simulink model "Communication_Testing"  (R2024a)
settings: Solver=FixedStepAuto  StartTime=0.0  StopTime=100  RelTol=1e-3  EnableMultiTasking=on
undefined symbols (not defined in the file or in its folder): CAN, FD
libraries: stmutilitieslib x29, simulink x25, stm32blockslib x11, canfdmsglib x7, stm32h7xxblockslib x3, dspstat3 x3, slpidlib x2
(part 2 of 2)

== system Communication_Testing/If Action Subsystem7 ==
  In1 : Inport
  Action Port : ActionPort  ActionPortLabel=case [ 235 ]:
  Out1 : Outport
  wires:
  In1/1 -> Out1/1

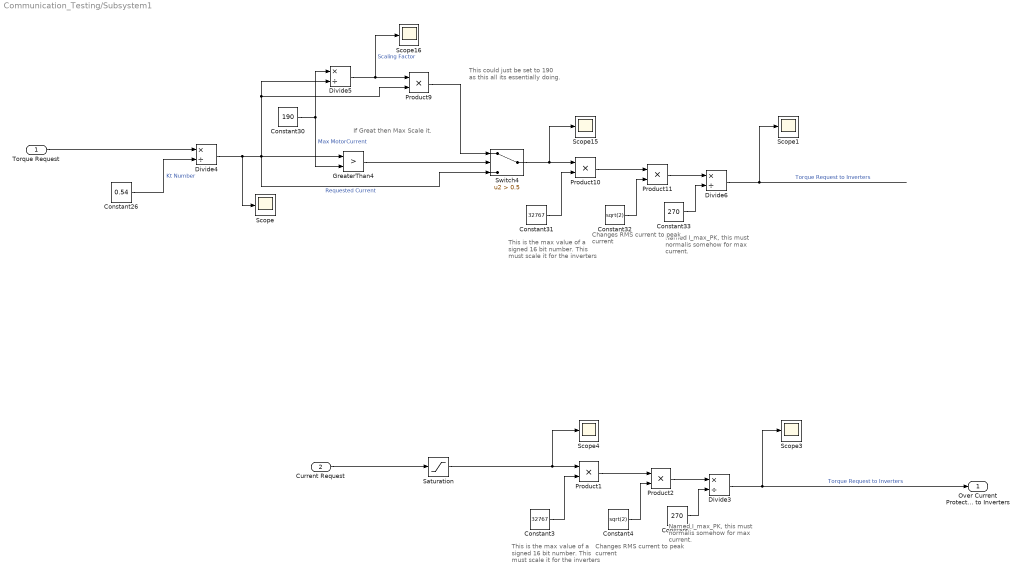
== system Communication_Testing/Subsystem1 ==
  note: This could just be set to 190 as this all its essentially doing.
  note: Named I_max_PK, this must normalis somehow for max current.
  note: Changes RMS current to peak current
  note: This is the max value of a signed 16 bit number. This must scale it for the inverters
  note: If Great then Max Scale it.
  note: Changes RMS current to peak current
  note: This is the max value of a signed 16 bit number. This must scale it for the inverters
  note: Named I_max_PK, this must normalis somehow for max current.
  Torque Request : Inport
  Current Request : Inport  Port=2
  Constant26 : Constant  Value=0.54
  Constant3 : Constant  Value=32767
  Constant30 : Constant  Value=190
  Constant31 : Constant  Value=32767
  Constant32 : Constant  Value=sqrt(2)
  Constant33 : Constant  Value=270
  Constant4 : Constant  Value=sqrt(2)
  Constant5 : Constant  Value=270
  Divide{3..6} (4 alike) : Product  Inputs=*/
  GreaterThan4 : RelationalOperator  Operator=>  OutDataTypeStr=boolean  RndMeth=Simplest  InputSameDT=off
  Product{1..2,9..11} (5 alike) : Product
  Saturation : Saturate  UpperLimit=190  LowerLimit=0
  Scope{,1,3..4,15..16} (6 alike) : Scope
  Switch4 : Switch  Criteria=u2 > Threshold  Threshold=0.5  SaturateOnIntegerOverflow=off  InputSameDT=off
  Over Current Protected Torque Request to Inverters : Outport
  wires:
  Constant31/1 -> Product10/2
  Product10/1 -> Product11/1
  Constant33/1 -> Divide6/2
  GreaterThan4/1 -> Switch4/2
  Divide5/1 -> Scope16/1, Product9/1  "Scaling Factor"
  Constant30/1 -> Divide5/1, GreaterThan4/2  "Max MotorCurrent"
  Product9/1 -> Switch4/1
  Divide4/1 -> Scope/1, Product9/2, Divide5/2, Switch4/3, GreaterThan4/1  "Requested Current"
  Constant26/1 -> Divide4/2  "Kt Number"
  Switch4/1 -> Product10/1, Scope15/1
  Constant32/1 -> Product11/2
  Product11/1 -> Divide6/1
  Torque Request/1 -> Divide4/1
  Divide6/1 -> Scope1/1  "Torque Request to Inverters"
  Product1/1 -> Product2/1
  Saturation/1 -> Product1/1, Scope4/1
  Divide3/1 -> Over Current Protected Torque Request to Inverters/1, Scope3/1  "Torque Request to Inverters"
  Constant4/1 -> Product2/2
  Constant5/1 -> Divide3/2
  Constant3/1 -> Product1/2
  Product2/1 -> Divide3/1
  Current Request/1 -> Saturation/1

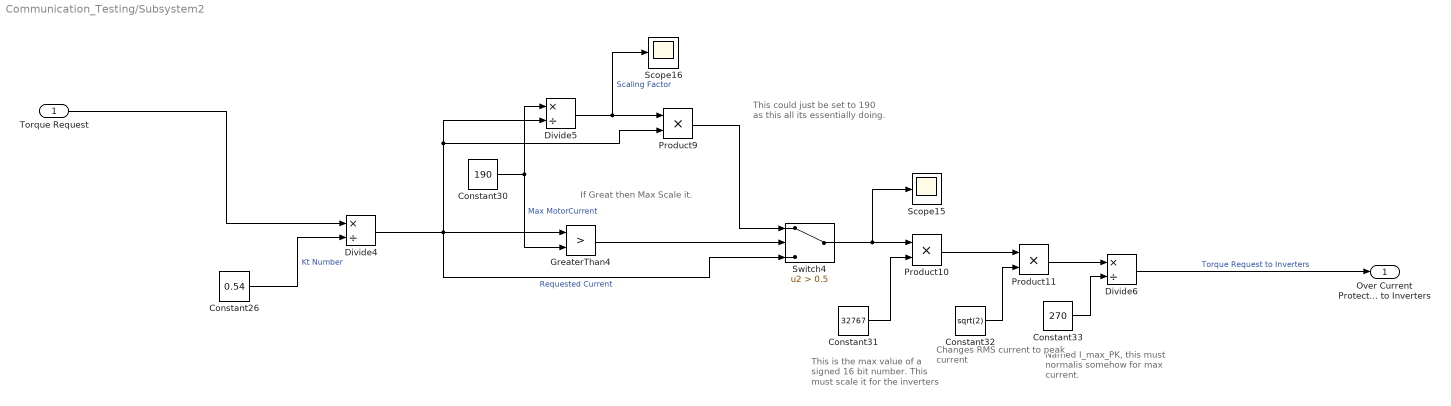
== system Communication_Testing/Subsystem2 ==
  note: This could just be set to 190 as this all its essentially doing.
  note: Named I_max_PK, this must normalis somehow for max current.
  note: Changes RMS current to peak current
  note: This is the max value of a signed 16 bit number. This must scale it for the inverters
  note: If Great then Max Scale it.
  Torque Request : Inport
  Constant26 : Constant  Value=0.54
  Constant30 : Constant  Value=190
  Constant31 : Constant  Value=32767
  Constant32 : Constant  Value=sqrt(2)
  Constant33 : Constant  Value=270
  Divide4 : Product  Inputs=*/
  Divide5 : Product  Inputs=*/
  Divide6 : Product  Inputs=*/
  GreaterThan4 : RelationalOperator  Operator=>  OutDataTypeStr=boolean  RndMeth=Simplest  InputSameDT=off
  Product10 : Product
  Product11 : Product
  Product9 : Product
  Scope15 : Scope
  Scope16 : Scope
  Switch4 : Switch  Criteria=u2 > Threshold  Threshold=0.5  SaturateOnIntegerOverflow=off  InputSameDT=off
  Over Current Protected Torque Request to Inverters : Outport
  wires:
  Constant31/1 -> Product10/2
  Product10/1 -> Product11/1
  Constant33/1 -> Divide6/2
  GreaterThan4/1 -> Switch4/2
  Divide5/1 -> Scope16/1, Product9/1  "Scaling Factor"
  Constant30/1 -> Divide5/1, GreaterThan4/2  "Max MotorCurrent"
  Product9/1 -> Switch4/1
  Divide4/1 -> Product9/2, Divide5/2, Switch4/3, GreaterThan4/1  "Requested Current"
  Constant26/1 -> Divide4/2  "Kt Number"
  Switch4/1 -> Product10/1, Scope15/1
  Constant32/1 -> Product11/2
  Product11/1 -> Divide6/1
  Torque Request/1 -> Divide4/1
  Divide6/1 -> Over Current Protected Torque Request to Inverters/1  "Torque Request to Inverters"

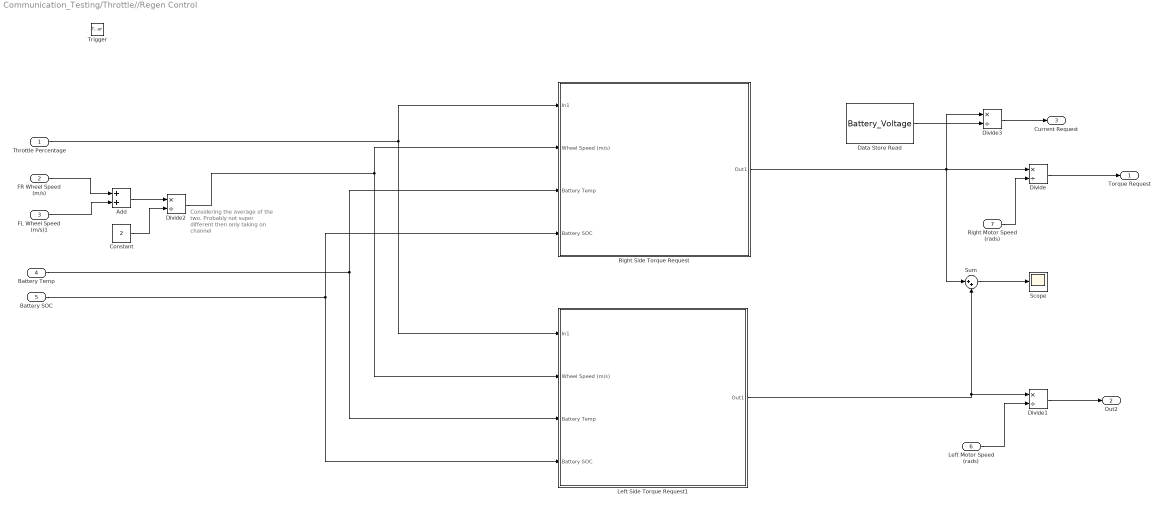
== system Communication_Testing/Throttle//Regen Control ==
  note: Considering the average of the two. Probably not super different then only taking on channel
  Throttle Percentage : Inport
  FR Wheel Speed (m/s) : Inport  Port=2
  FL Wheel Speed (m/s)1 : Inport  Port=3
  Battery Temp : Inport  Port=4
  Battery SOC : Inport  Port=5
  Left Motor Speed (rads) : Inport  Port=6
  Right Motor Speed (rads) : Inport  Port=7
  Trigger : TriggerPort  TriggerType=function-call  VariantControl=(inherit)
  Add : Sum
  Constant : Constant  Value=2
  Data Store Read : DataStoreRead  DataStoreName=Battery_Voltage  IndexOptions=Index vector (dialog)  Indices=1  OutputSizes=1
  Divide{,1..3} (4 alike) : Product  Inputs=*/
  Left Side Torque Request1 : Subsystem
  Right Side Torque Request : Subsystem
  Scope : Scope
  Sum : Sum  Inputs=|++
  Torque Request : Outport
  Out2 : Outport  Port=2
  Current Request : Outport  Port=3
  wires:
  Right Side Torque Request/1(Out1) -> Divide3/1, Divide/1, Sum/1
  Divide/1 -> Torque Request/1
  Left Motor Speed (rads)/1 -> Divide1/2
  Sum/1 -> Scope/1
  Left Side Torque Request1/1(Out1) -> Divide1/1, Sum/2
  Divide1/1 -> Out2/1
  Throttle Percentage/1 -> Left Side Torque Request1/1(In1), Right Side Torque Request/1(In1)
  Right Motor Speed (rads)/1 -> Divide/2
  Divide2/1 -> Left Side Torque Request1/2(Wheel Speed (m/s)), Right Side Torque Request/2(Wheel Speed (m/s))
  Battery Temp/1 -> Right Side Torque Request/3(Battery Temp), Left Side Torque Request1/3(Battery Temp)
  Battery SOC/1 -> Right Side Torque Request/4(Battery SOC), Left Side Torque Request1/4(Battery SOC)
  FR Wheel Speed (m/s)/1 -> Add/1
  FL Wheel Speed (m/s)1/1 -> Add/2
  Add/1 -> Divide2/1
  Constant/1 -> Divide2/2
  Data Store Read/1 -> Divide3/2
  Divide3/1 -> Current Request/1

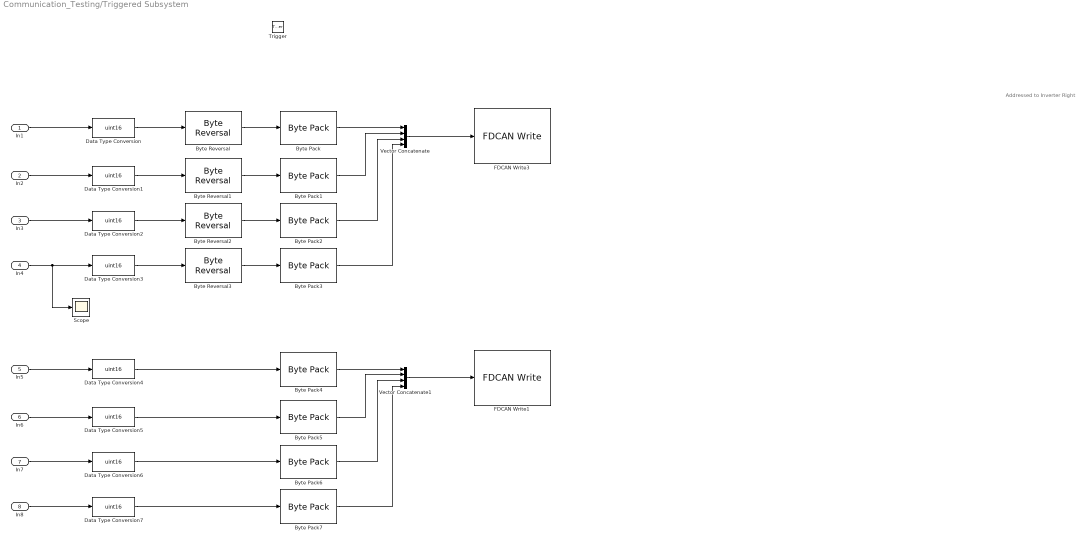
== system Communication_Testing/Triggered Subsystem ==
  note: Addressed to Inverter Right
  In1 : Inport
  In2 : Inport  Port=2
  In3 : Inport  Port=3
  In4 : Inport  Port=4
  In5 : Inport  Port=5
  In6 : Inport  Port=6
  In7 : Inport  Port=7
  In8 : Inport  Port=8
  Trigger : TriggerPort  TriggerType=function-call  VariantControl=(inherit)
  Byte Pack{,1..7} (8 alike) : stmutilitieslib/Byte Pack  datatypes={'uint16'}  byteAlign=1  blockPlatform=stm32f4discovery
  Byte Reversal{,1..3} (4 alike) : stmutilitieslib/Byte Reversal  numInp=1  blockPlatform=stm32f4discovery
  Data Type Conversion{,1..7} (8 alike) : DataTypeConversion  OutDataTypeStr=uint16  SaturateOnIntegerOverflow=off  RndMeth=Floor
  FDCAN Write1 : stm32blockslib/FDCAN Write  FDCANModule=FDCAN2  BlockMode=Transmit  OperationReadMode=Data  OperationWriteMode=Data  ReadSource=FIFO 0  BufferNumber=0  OutputTypeReadMode=Unpacked  DataFormatWriteMode=Raw data  CANFrameType=CAN  IdentifierTypeVia=Dialog  IdentifierType=Standard (11-bit identifier)  IdentifierVia=Dialog  Identifier=9  DataLengthVia=Dialog  DataLength=8  OutputIdType=off  IsBitRateSwitchingEnabled=off  TransmitRemoteFrame=off  OutputFrameType=off  OutputBRS=off  OutputRemoteFrame=off  OutputTxFifoLevel=off  OutputRxFifoLevel=off  OutputStatus=off  Timeout=1  SampleTime=-1
      settings: LibrarySourceBlock=stm32l5xxblockslib/FDCAN Write
  FDCAN Write3 : stm32blockslib/FDCAN Write  FDCANModule=FDCAN2  BlockMode=Transmit  OperationReadMode=Data  OperationWriteMode=Data  ReadSource=FIFO 0  BufferNumber=0  OutputTypeReadMode=Unpacked  DataFormatWriteMode=Raw data  CANFrameType=CAN  IdentifierTypeVia=Dialog  IdentifierType=Standard (11-bit identifier)  IdentifierVia=Dialog  Identifier=8  DataLengthVia=Dialog  DataLength=8  OutputIdType=off  IsBitRateSwitchingEnabled=off  TransmitRemoteFrame=off  OutputFrameType=off  OutputBRS=off  OutputRemoteFrame=off  OutputTxFifoLevel=off  OutputRxFifoLevel=off  OutputStatus=off  Timeout=1  SampleTime=-1
      settings: LibrarySourceBlock=stm32l5xxblockslib/FDCAN Write
  Scope : Scope
  Vector Concatenate : Concatenate  NumInputs=4
  Vector Concatenate1 : Concatenate  NumInputs=4
  wires:
  Byte Reversal/1 -> Byte Pack/1
  Byte Pack/1 -> Vector Concatenate/1
  Data Type Conversion/1 -> Byte Reversal/1
  In1/1 -> Data Type Conversion/1
  Byte Pack1/1 -> Vector Concatenate/2
  Byte Reversal1/1 -> Byte Pack1/1
  Data Type Conversion1/1 -> Byte Reversal1/1
  Byte Pack2/1 -> Vector Concatenate/3
  Byte Reversal2/1 -> Byte Pack2/1
  Data Type Conversion2/1 -> Byte Reversal2/1
  Byte Pack3/1 -> Vector Concatenate/4
  Byte Reversal3/1 -> Byte Pack3/1
  Data Type Conversion3/1 -> Byte Reversal3/1
  In2/1 -> Data Type Conversion1/1
  In3/1 -> Data Type Conversion2/1
  In4/1 -> Scope/1, Data Type Conversion3/1
  Vector Concatenate/1 -> FDCAN Write3/1
  Byte Pack6/1 -> Vector Concatenate1/3
  Data Type Conversion7/1 -> Byte Pack7/1
  Vector Concatenate1/1 -> FDCAN Write1/1
  Byte Pack5/1 -> Vector Concatenate1/2
  Byte Pack7/1 -> Vector Concatenate1/4
  Byte Pack4/1 -> Vector Concatenate1/1
  Data Type Conversion5/1 -> Byte Pack5/1
  Data Type Conversion6/1 -> Byte Pack6/1
  Data Type Conversion4/1 -> Byte Pack4/1
  In8/1 -> Data Type Conversion7/1
  In7/1 -> Data Type Conversion6/1
  In6/1 -> Data Type Conversion5/1
  In5/1 -> Data Type Conversion4/1

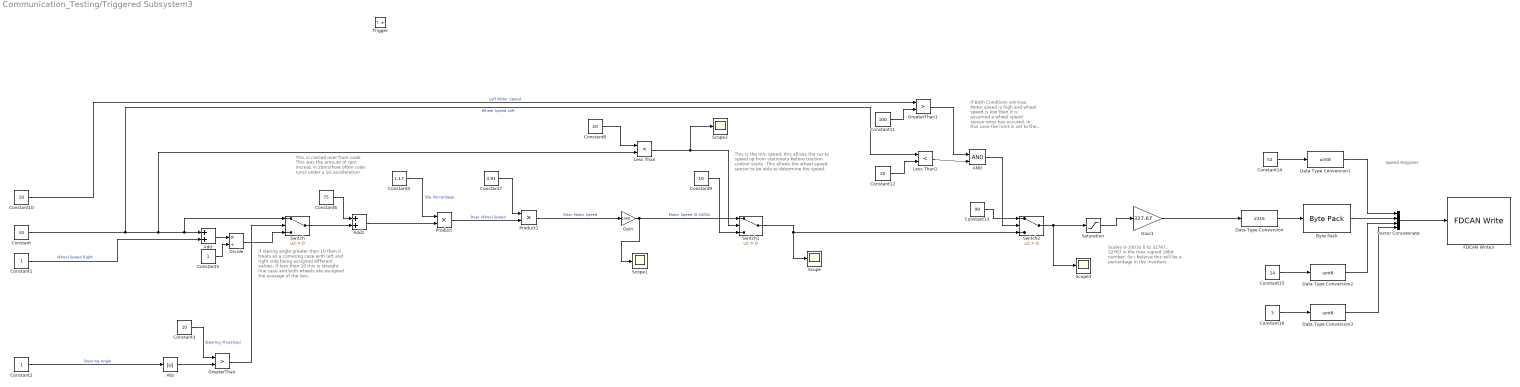
== system Communication_Testing/Triggered Subsystem3 ==
  note: This is the min speed, this allows the car to speed up from stationary before traction control starts, This allows the wheel speed sensor to be able to determine the speed.
  note: Scales 0-100 to 0 to 32767, 32767 is the max signed 16bit number, So i beleive this will be a percentage in the inverters
  note: If Both Conditons are true. Motor speed is high and wheel speed is low then it is assumed a wheel speed sensor error has occured. In this case the limit is set to the maximum.
  note: This is carried over from code. This was the amount of rpm increas in 20ms(how often code runs) under a 1G acceleration
  note: Speed Register
  note: if stering angle greater then 10 then it treats as a cornering case with left and right side being assigned different values. If less then 10 this is straight line case and both wheels are assigned the average of the two.
  Trigger : TriggerPort  TriggerType=function-call  VariantControl=(inherit)
  AND : Logic  IconShape=distinctive  AllPortsSameDT=off  OutDataTypeStr=boolean
  Abs : Abs  SaturateOnIntegerOverflow=off
  Add : Sum
  Add1 : Sum
  Byte Pack : stmutilitieslib/Byte Pack  datatypes={'int16'}  byteAlign=1  blockPlatform=stm32f4discovery
  Constant{,3,9..10} (4 alike) : Constant  Value=10
  Constant1 : Constant
  Constant11 : Constant  Value=100
  Constant12 : Constant  Value=20
  Constant13 : Constant  Value=99
  Constant14 : Constant  Value=52
  Constant15 : Constant  Value=14
  Constant16 : Constant  Value=3
  Constant2 : Constant
  Constant4 : Constant  Value=1.17
  Constant5 : Constant
  Constant6 : Constant  Value=75
  Constant7 : Constant  Value=3.91
  Constant8 : Constant  Value=20
  Data Type Conversion : DataTypeConversion  OutDataTypeStr=int16  SaturateOnIntegerOverflow=off  RndMeth=Floor
  Data Type Conversion1 : DataTypeConversion  OutDataTypeStr=uint8  SaturateOnIntegerOverflow=off  RndMeth=Floor
  Data Type Conversion2 : DataTypeConversion  OutDataTypeStr=uint8  SaturateOnIntegerOverflow=off  RndMeth=Floor
  Data Type Conversion3 : DataTypeConversion  OutDataTypeStr=uint8  SaturateOnIntegerOverflow=off  RndMeth=Floor
  Divide : Product  Inputs=*/
  FDCAN Write3 : stm32blockslib/FDCAN Write  FDCANModule=FDCAN2  BlockMode=Transmit  OperationReadMode=Data  OperationWriteMode=Data  ReadSource=FIFO 0  BufferNumber=0  OutputTypeReadMode=Unpacked  DataFormatWriteMode=Raw data  CANFrameType=CAN  IdentifierTypeVia=Dialog  IdentifierType=Standard (11-bit identifier)  IdentifierVia=Dialog  Identifier=210  DataLengthVia=Dialog  DataLength=5  OutputIdType=off  IsBitRateSwitchingEnabled=off  TransmitRemoteFrame=off  OutputFrameType=off  OutputBRS=off  OutputRemoteFrame=off  OutputTxFifoLevel=off  OutputRxFifoLevel=off  OutputStatus=off  Timeout=1  SampleTime=-1
      settings: LibrarySourceBlock=stm32l5xxblockslib/FDCAN Write
  Gain : Gain  Gain=1/60
  Gain1 : Gain  Gain=327.67
  GreaterThan : RelationalOperator  Operator=>  OutDataTypeStr=boolean  RndMeth=Simplest  InputSameDT=off
  GreaterThan1 : RelationalOperator  Operator=>  OutDataTypeStr=boolean  RndMeth=Simplest  InputSameDT=off
  Less Than : RelationalOperator  Operator=<  OutDataTypeStr=boolean  RndMeth=Simplest  InputSameDT=off
  Less Than1 : RelationalOperator  Operator=<  OutDataTypeStr=boolean  RndMeth=Simplest  InputSameDT=off
  Product : Product
  Product1 : Product
  Saturation : Saturate  UpperLimit=99  LowerLimit=0
  Scope{,1..3} (4 alike) : Scope
  Switch : Switch  Criteria=u2 > Threshold  SaturateOnIntegerOverflow=off  InputSameDT=off
  Switch1 : Switch  Criteria=u2 > Threshold  SaturateOnIntegerOverflow=off  InputSameDT=off
  Switch2 : Switch  Criteria=u2 > Threshold  SaturateOnIntegerOverflow=off  InputSameDT=off
  Vector Concatenate : Concatenate  NumInputs=4
  wires:
  Data Type Conversion/1 -> Byte Pack/1
  Switch2/1 -> Scope3/1, Saturation/1
  Less Than1/1 -> AND/2
  Gain1/1 -> Data Type Conversion/1
  Constant13/1 -> Switch2/1
  Data Type Conversion1/1 -> Vector Concatenate/1
  AND/1 -> Switch2/2
  Switch1/1 -> Switch2/3, Scope/1
  Data Type Conversion2/1 -> Vector Concatenate/3
  GreaterThan1/1 -> AND/1
  Constant8/1 -> Less Than/1
  Saturation/1 -> Gain1/1
  Constant11/1 -> GreaterThan1/2
  Less Than/1 -> Switch1/2, Scope2/1
  Gain/1 -> Switch1/1, Scope1/1  "Motor Speed (0-100%)"
  Constant16/1 -> Data Type Conversion3/1
  Product1/1 -> Gain/1  "Rear Motor Speed"
  Divide/1 -> Switch/3
  Constant15/1 -> Data Type Conversion2/1
  Add1/1 -> Product/2
  Constant9/1 -> Switch1/3
  Constant2/1 -> Abs/1  "Steering Angle"
  Constant10/1 -> GreaterThan1/1  "Left Motor Speed"
  Add/1 -> Divide/1
  Constant4/1 -> Product/1  "Slip Percentage"
  Product/1 -> Product1/2  "Rear Wheel Speed"
  Constant12/1 -> Less Than1/2
  Constant5/1 -> Divide/2
  Constant3/1 -> GreaterThan/1  "Steering Threshold"
  Byte Pack/1 -> Vector Concatenate/2
  Switch/1 -> Add1/2
  Constant7/1 -> Product1/1
  Constant1/1 -> Add/2  "Wheel Speed Right"
  GreaterThan/1 -> Switch/2
  Constant6/1 -> Add1/1
  Constant14/1 -> Data Type Conversion1/1
  Constant/1 -> Less Than1/1, Less Than/2, Switch/1, Add/1  "Wheel Speed Left"
  Abs/1 -> GreaterThan/2
  Data Type Conversion3/1 -> Vector Concatenate/4
  Vector Concatenate/1 -> FDCAN Write3/1

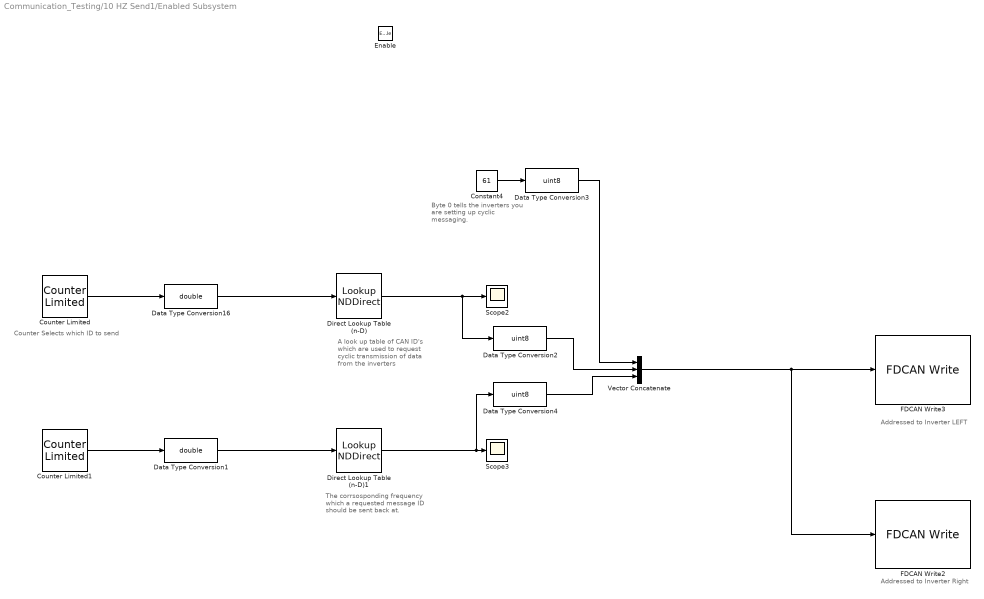
== system Communication_Testing/10 HZ Send1/Enabled Subsystem ==
  note: The corrsosponding frequency which a requested message ID should be sent back at.
  note: A look up table of CAN ID's which are used to request cyclic transmission of data from the inverters
  note: Byte 0 tells the inverters you are setting up cyclic messaging.
  note: Addressed to Inverter LEFT
  note: Counter Selects which ID to send
  note: Addressed to Inverter Right
  Enable : EnablePort
  Constant4 : Constant  Value=61
  Counter Limited : simulink/Sources/Counter Limited  uplimit=5  tsamp=-1
  Counter Limited1 : simulink/Sources/Counter Limited  uplimit=5  tsamp=-1
  Data Type Conversion1 : DataTypeConversion  OutDataTypeStr=double  SaturateOnIntegerOverflow=off  RndMeth=Floor
  Data Type Conversion16 : DataTypeConversion  OutDataTypeStr=double  SaturateOnIntegerOverflow=off  RndMeth=Floor
  Data Type Conversion2 : DataTypeConversion  OutDataTypeStr=uint8  SaturateOnIntegerOverflow=off  RndMeth=Floor
  Data Type Conversion3 : DataTypeConversion  OutDataTypeStr=uint8  SaturateOnIntegerOverflow=off  RndMeth=Floor
  Data Type Conversion4 : DataTypeConversion  OutDataTypeStr=uint8  SaturateOnIntegerOverflow=off  RndMeth=Floor
  Direct Lookup Table (n-D) : LookupNDDirect  NumberOfTableDimensions=1  Table=[235 74 168 73 95 138]
  Direct Lookup Table (n-D)1 : LookupNDDirect  NumberOfTableDimensions=1  Table=[235 74 168 73 95 138]
  FDCAN Write2 : stm32blockslib/FDCAN Write  FDCANModule=FDCAN2  BlockMode=Transmit  OperationReadMode=Data  OperationWriteMode=Data  ReadSource=FIFO 0  BufferNumber=0  OutputTypeReadMode=Unpacked  DataFormatWriteMode=Raw data  CANFrameType=CAN  IdentifierTypeVia=Dialog  IdentifierType=Standard (11-bit identifier)  IdentifierVia=Dialog  Identifier=529  DataLengthVia=Dialog  DataLength=3  OutputIdType=off  IsBitRateSwitchingEnabled=off  TransmitRemoteFrame=off  OutputFrameType=off  OutputBRS=off  OutputRemoteFrame=off  OutputTxFifoLevel=off  OutputRxFifoLevel=off  OutputStatus=off  Timeout=1  SampleTime=-1
      settings: LibrarySourceBlock=stm32l5xxblockslib/FDCAN Write
  FDCAN Write3 : stm32blockslib/FDCAN Write  FDCANModule=FDCAN2  BlockMode=Transmit  OperationReadMode=Data  OperationWriteMode=Data  ReadSource=FIFO 0  BufferNumber=0  OutputTypeReadMode=Unpacked  DataFormatWriteMode=Raw data  CANFrameType=CAN  IdentifierTypeVia=Dialog  IdentifierType=Standard (11-bit identifier)  IdentifierVia=Dialog  Identifier=528  DataLengthVia=Dialog  DataLength=3  OutputIdType=off  IsBitRateSwitchingEnabled=off  TransmitRemoteFrame=off  OutputFrameType=off  OutputBRS=off  OutputRemoteFrame=off  OutputTxFifoLevel=off  OutputRxFifoLevel=off  OutputStatus=off  Timeout=1  SampleTime=-1
      settings: LibrarySourceBlock=stm32l5xxblockslib/FDCAN Write
  Scope2 : Scope
  Scope3 : Scope
  Vector Concatenate : Concatenate  NumInputs=3
  wires:
  Direct Lookup Table (n-D)1/1 -> Data Type Conversion4/1, Scope3/1
  Data Type Conversion1/1 -> Direct Lookup Table (n-D)1/1
  Data Type Conversion16/1 -> Direct Lookup Table (n-D)/1
  Direct Lookup Table (n-D)/1 -> Data Type Conversion2/1, Scope2/1
  Counter Limited1/1 -> Data Type Conversion1/1
  Counter Limited/1 -> Data Type Conversion16/1
  Vector Concatenate/1 -> FDCAN Write2/1, FDCAN Write3/1
  Data Type Conversion3/1 -> Vector Concatenate/1
  Data Type Conversion4/1 -> Vector Concatenate/3
  Data Type Conversion2/1 -> Vector Concatenate/2
  Constant4/1 -> Data Type Conversion3/1

== system Communication_Testing/Function-Call Subsystem/If Action Subsystem1 ==
  In1 : Inport
  Action Port : ActionPort  ActionPortLabel=case [ 138 ]:
  Out1 : Outport
  wires:
  In1/1 -> Out1/1

== system Communication_Testing/Function-Call Subsystem/If Action Subsystem10 ==
  In1 : Inport
  Action Port : ActionPort  ActionPortLabel=case [ 168 ]:
  Out1 : Outport
  wires:
  In1/1 -> Out1/1

== system Communication_Testing/Function-Call Subsystem/If Action Subsystem11 ==
  In1 : Inport
  Action Port : ActionPort  ActionPortLabel=case [ 74 ]:
  Out1 : Outport
  wires:
  In1/1 -> Out1/1

== system Communication_Testing/Function-Call Subsystem/If Action Subsystem12 ==
  In1 : Inport
  Action Port : ActionPort  ActionPortLabel=case [ 235 ]:
  Out1 : Outport
  wires:
  In1/1 -> Out1/1

== system Communication_Testing/Function-Call Subsystem/If Action Subsystem2 ==
  In1 : Inport
  Action Port : ActionPort  ActionPortLabel=case [ 95 ]:
  Out1 : Outport
  wires:
  In1/1 -> Out1/1

== system Communication_Testing/Function-Call Subsystem/If Action Subsystem3 ==
  In1 : Inport
  Action Port : ActionPort  ActionPortLabel=case [ 73 ]:
  Out1 : Outport
  wires:
  In1/1 -> Out1/1

== system Communication_Testing/Function-Call Subsystem/If Action Subsystem4 ==
  In1 : Inport
  Action Port : ActionPort  ActionPortLabel=case [ 168 ]:
  Out1 : Outport
  wires:
  In1/1 -> Out1/1

== system Communication_Testing/Function-Call Subsystem/If Action Subsystem5 ==
  In1 : Inport
  Action Port : ActionPort  ActionPortLabel=case [ 74 ]:
  Out1 : Outport
  wires:
  In1/1 -> Out1/1

== system Communication_Testing/Function-Call Subsystem/If Action Subsystem6 ==
  In1 : Inport
  Action Port : ActionPort  ActionPortLabel=case [ 235 ]:
  Out1 : Outport
  wires:
  In1/1 -> Out1/1

== system Communication_Testing/Function-Call Subsystem/If Action Subsystem7 ==
  In1 : Inport
  Action Port : ActionPort  ActionPortLabel=case [ 138 ]:
  Out1 : Outport
  wires:
  In1/1 -> Out1/1

== system Communication_Testing/Function-Call Subsystem/If Action Subsystem8 ==
  In1 : Inport
  Action Port : ActionPort  ActionPortLabel=case [ 95 ]:
  Out1 : Outport
  wires:
  In1/1 -> Out1/1

== system Communication_Testing/Function-Call Subsystem/If Action Subsystem9 ==
  In1 : Inport
  Action Port : ActionPort  ActionPortLabel=case [ 73 ]:
  Out1 : Outport
  wires:
  In1/1 -> Out1/1

== system Communication_Testing/Function-Call Subsystem2/Subsystem ==
  Constant2 : Constant
  Out1 : Outport
  wires:
  Constant2/1 -> Out1/1

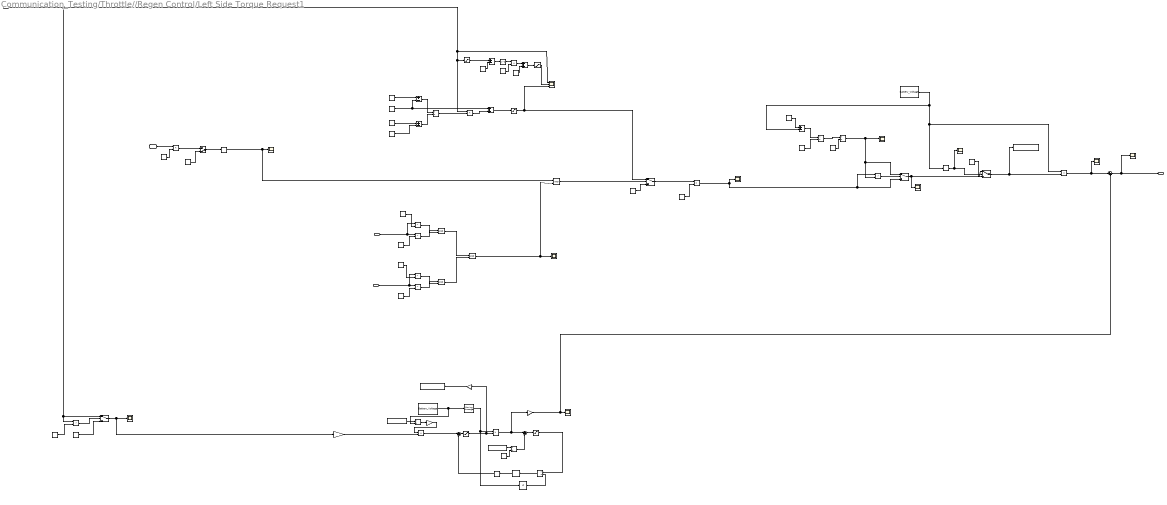
== system Communication_Testing/Throttle//Regen Control/Left Side Torque Request1 ==
  note: Divide by two as the global power is the power limit for the whole vehicle, then need the left and right side power limits
  note: Halveing as this is the permissable for left/right side inverter
  note: If Conditions are not fulfilled charge current is set to zero
  note: This function was made in Desmos. Adjusted to meet cross over and start of rise
  note: Throttle pedal to regen percentage request
  note: Power Limiting to maintatin Power Limit of Less then 80 Kw
  note: Inverting as this is a discharge current
  note: throttle output enabled when less then 20% actuation, this will be used for regen
  note: If Battery Voltage greater then 590 Charge Current is set to zero
  note: Throttle Mapping to Regen Percentage
  note: Limiting the input range
  note: Speed Threshold, Regen enabled above 5km/h
  note: Max Charge Current, Regen is scalled 0-100%. Current wants to be 0 -130 amps, therfore scale by 1.3. 600V*130amps = 70kw, Then divide by two for left and right motor Control
  note: Hysterisies Control
  note: Inverting as this is a discharge current
  note: Battery Checks
  note: This is the threshold for when drive torque is requested, Regen is requested for less then 20%, and throttle is applied for greater then 22%, This gives a 2% deadband
  note: If Requested Charge current is greater then permissable charge current then switch to permisable
  In1 : Inport
  Wheel Speed (m/s) : Inport  Port=2
  Battery Temp : Inport  Port=3
  Battery SOC : Inport  Port=4
  AND{,1..3} (4 alike) : Logic  IconShape=distinctive  AllPortsSameDT=off  OutDataTypeStr=boolean
  Add2 : Sum
  Add3 : Sum
  Compare To Constant : simulink/Logic and Bit Operations/Compare To Constant  relop=>  const=5  OutDataTypeStr=boolean
  Constant : Constant  Value=2
  Constant{7,10..11,21,28} (5 alike) : Constant  Value=0
  Constant12 : Constant  Value=6
  Constant15 : Constant  Value=0.01
  Constant16 : Constant  Value=50
  Constant17 : Constant  Value=10
  Constant18 : Constant  Value=90
  Constant19 : Constant  Value=5
  Constant2 : Constant  Value=3.6
  Constant20 : Constant  Value=580
  Constant26 : Constant  Value=2
  Constant27 : Constant  Value=22
  Constant3 : Constant  Value=20
  Constant4 : Constant  Value=10
  Constant5 : Constant  Value=100
  Constant6 : Constant  Value=20
  Constant9 : Constant  Value=0.25
  Data Store Read : DataStoreRead  DataStoreName=Battery_Voltage  IndexOptions=Index vector (dialog)  Indices=1  OutputSizes=1
  Data Store Read1 : DataStoreRead  DataStoreName=Battery_Voltage  IndexOptions=Index vector (dialog)  Indices=1  OutputSizes=1
  Data Store Read2 : DataStoreRead  DataStoreName=Global_Power_Limit  IndexOptions=Index vector (dialog)  Indices=1  OutputSizes=1
  Data Store Read3 : DataStoreRead  DataStoreName=Global_Power_Limit  IndexOptions=Index vector (dialog)  Indices=1  OutputSizes=1
  Data Store Write : DataStoreWrite  DataStoreName=Left_Sim_Regen_Current  IndexOptions=Index vector (dialog)  Indices=1  OutputSizes=1
  Data Store Write1 : DataStoreWrite  DataStoreName=Left_Sim_Discharge_Current  IndexOptions=Index vector (dialog)  Indices=1  OutputSizes=1
  Discrete PID Controller1 : slpidlib/PID Controller  Controller=PID  Form=Parallel  TimeDomain=Discrete-time  UseExternalTs=off  SampleTime=-1  IntegratorMethod=Forward Euler  FilterMethod=Forward Euler  ControllerParametersSource=internal  P=0.000544217300579932  I=0.544217300579932  UseKiTs=on  D=0  UseExternalDerivativeSource=off  N=100  UseFilter=on  TunerSelectOption=Transfer Function Based (PID Tuner App)  InitialConditionSource=internal  InitialConditionForIntegrator=10  InitialConditionForFilter=0  DifferentiatorICPrevScaledInput=0  ExternalReset=none  TrackingMode=off  Kt=1  LimitOutput=off  SatLimitsSource=internal  UpperSaturationLimit=inf  LowerSaturationLimit=-inf  LinearizeAsGain=off  AntiWindupMode=none  Kb=1  LimitIntegrator=off  UpperIntegratorSaturationLimit=inf  LowerIntegratorSaturationLimit=-inf  POutMin=[]  POutMax=[]  IOutMin=[]  IOutMax=[]  DOutMin=[]  DOutMax=[]  NOutMin=[]  NOutMax=[]  SumOutMin=[]  SumOutMax=[]  SaturationOutMin=[]  SaturationOutMax=[]  PParamMin=[]  PParamMax=[]  IParamMin=[]  IParamMax=[]  DParamMin=[]  DParamMax=[]  NParamMin=[]  NParamMax=[]  KbParamMin=[]  KbParamMax=[]  KtParamMin=[]  KtParamMax=[]  KbOutMin=[]  KbOutMax=[]  KtOutMin=[]  KtOutMax=[]  IntegratorOutMin=[]  IntegratorOutMax=[]  FilterOutMin=[]  FilterOutMax=[]  SumI1OutMin=[]  SumI1OutMax=[]  SumI2OutMin=[]  SumI2OutMax=[]  SumI3OutMin=[]  SumI3OutMax=[]  SumI4OutMin=[]  SumI4OutMax=[]  SumDOutMin=[]  SumDOutMax=[]  DifferentiatorOutMin=[]  DifferentiatorOutMax=[]  FilterDiffOutCoefMin=[]  FilterDiffOutCoefMax=[]  ReciprocalOutMin=[]  ReciprocalOutMax=[]  SumDenOutMin=[]  SumDenOutMax=[]  SumNumOutMin=[]  SumNumOutMax=[]  DivideOutMin=[]  DivideOutMax=[]  UdiffTsProdOutMin=[]  UdiffTsProdOutMax=[]  NTsProdOutMin=[]  NTsProdOutMax=[]  UintegralTsProdOutMin=[]  UintegralTsProdOutMax=[]  UngainTsProdOutMin=[]  UngainTsProdOutMax=[]  ClampingZeroOutDataTypeStr=Inherit: Inherit via back propagation  ClampingZeroOutMin=[]  ClampingZeroOutMax=[]  FilterDenConstantOutDataTypeStr=Inherit: Inherit via back propagation  FilterDenConstantOutMin=[]  FilterDenConstantOutMax=[]  PCopyOutDataTypeStr=Inherit: Inherit via back propagation  PCopyOutMin=[]  PCopyOutMax=[]  NCopyOutDataTypeStr=Inherit: Inherit via back propagation  NCopyOutMin=[]  NCopyOutMax=[]  IntegratorContinuousStateAttributes=''  IntegratorStateMustResolveToSignalObject=off  IntegratorRTWStateStorageClass=Auto  FilterContinuousStateAttributes=''  FilterStateMustResolveToSignalObject=off  FilterRTWStateStorageClass=Auto  ParallelPVariant=InternalParameters  IdealPVariant=Disabled  IVariant=InternalParameters  DVariant=InternalParameters  IntegratorVariant=Discrete  SatVariant=Disabled  AWVariant=Passthrough  PCopyVariant=Disabled  TRVariant=Disabled  FdbkBlocksVariant=Forward  IdealPFdbkVariant=Disabled  SatFdbkVariant=Disabled  DerivativeFilterVariant=ForwardEulerFilter  NVariant=InternalParameters  NCopyVariant=Disabled  FilterICVariant=InternalICsFilter  IntegratorICVariant=InternalICs  ExternalResetVariant=Disabled  TRSumVariant=Passthrough  SumFdbkVariant=Disabled  SumVariant=Sum_PID  TsampFilterVariant=InternalTs  TsampNgainVariant=Passthrough  TsampIntegralVariant=Disabled_SignalSpec  ExternalSaturationOutDataTypeStr=Inherit: Same as second input  DerivativeSourceVariant=ErrorSignal
      settings: LibrarySourceBlock=simulink/Discrete/Discrete PID Controller
  Divide{,1..5} (6 alike) : Product  Inputs=*/
  Gain : Gain  Gain=-1
  Gain1 : Gain  Gain=-1
  Gain2 : Gain  Gain=1/100
  Gain3 : Gain  Gain=1.1
  GreaterThan{,1..3} (4 alike) : RelationalOperator  Operator=>  OutDataTypeStr=boolean  RndMeth=Simplest  InputSameDT=off
  IC1 : InitialCondition  Value=600
  Less Than : RelationalOperator  Operator=<  OutDataTypeStr=boolean  RndMeth=Simplest  InputSameDT=off
  Less Than1 : RelationalOperator  Operator=<  OutDataTypeStr=boolean  RndMeth=Simplest  InputSameDT=off
  Manual Switch1 : ManualSwitch  CurrentSetting=0
  Memory1 : Memory  InitialCondition=14  InheritSampleTime=on
  Minus : Sum  Inputs=+-
  Moving Average : dspstat3/Moving Average  Method=Sliding window  ForgettingFactorPort=off  SpecifyWindowLength=on  WindowLength=10  OverlapLength=9  AllowArbitraryInputLength=off  ForgettingFactor=0.9  SimulateUsing=Interpreted execution
  Product{1..7} (7 alike) : Product
  Relay : Relay  OnSwitchValue=590  OffSwitchValue=585  OnOutputValue=0  OffOutputValue=1
  Saturation : Saturate  UpperLimit=100  LowerLimit=0
  Saturation1 : Saturate  UpperLimit=100  LowerLimit=0
  Saturation2 : Saturate  UpperLimit=20  LowerLimit=0
  Saturation3 : Saturate  UpperLimit=inf  LowerLimit=0
  Saturation5 : Saturate  UpperLimit=inf  LowerLimit=0
  Scale : Constant  Value=0.65
  Scope{,1,3,5,7..9,11,13..14} (10 alike) : Scope
  Scope2 : Scope  NumInputPorts=3
  Square : Math  Operator=square
  Subtract : Sum  Inputs=+-
  Subtract1 : Sum  Inputs=+-
  Subtract2 : Sum  Inputs=+-
  Sum : Sum  Inputs=|+-
  Sum1 : Sum  Inputs=|+-
  Sum3 : Sum  Inputs=|++
  Switch : Switch  Criteria=u2 > Threshold  SaturateOnIntegerOverflow=off  InputSameDT=off
  Switch1 : Switch  Criteria=u2 > Threshold  SaturateOnIntegerOverflow=off  InputSameDT=off
  Switch2 : Switch  Criteria=u2 > Threshold  Threshold=0.5  SaturateOnIntegerOverflow=off  InputSameDT=off
  Switch3 : Switch  Criteria=u2 > Threshold  SaturateOnIntegerOverflow=off  InputSameDT=off
  Out1 : Outport
  wires:
  Constant26/1 -> Divide4/2
  Product3/1 -> Add2/1
  Constant10/1 -> Add2/2
  Constant3/1 -> Subtract2/2
  AND/1 -> Switch/2
  Add3/1 -> Saturation/1  "Regen Request"
  GreaterThan2/1 -> Switch1/2
  Constant12/1 -> Manual Switch1/2
  GreaterThan1/1 -> AND2/1
  Constant21/1 -> Switch2/3
  In1/1 -> Switch3/1, GreaterThan3/1, Product2/1, Saturation2/1, Scope2/1  "Throttle Pedal"
  Constant11/1 -> Switch/3
  Switch3/1 -> Gain2/1, Scope14/1  "Throttle Percentage > 20"
  Product5/1 -> Sum1/1, Gain1/1  "Requested Discharge Power"
  Saturation/1 -> Switch/1, Scope2/3  "Linear Regen Map"
  Switch/1 -> Product4/1  "Requested Charge Current"
  Saturation1/1 -> Scope2/2  "Exponential Throttle Map"
  Gain1/1 -> Sum3/2, Scope5/1
  Constant27/1 -> GreaterThan3/2
  Constant20/1 -> Minus/1  "Max Battery Voltage using Regen"
  Constant5/1 -> Subtract/2, Add3/1  "Max Regen Percentage"
  Constant19/1 -> GreaterThan1/2  "Min Battery SOC"
  Subtract2/1 -> Square/1
  Product7/1 -> Scope13/1, Sum3/1  "Requested Charge Power"
  Subtract/1 -> Divide1/1
  Battery SOC/1 -> GreaterThan1/1, Less Than1/1  "Battery State of Charge"
  Moving Average/1 -> IC1/1, Product5/1
  Saturation3/1 -> Divide2/1  "Power Error"
  Manual Switch1/1 -> Compare To Constant/1
  Product1/1 -> Manual Switch1/1  "Speed (km/h)"
  Subtract1/1 -> Divide1/2
  Constant17/1 -> GreaterThan/2  "Min Battery Temp"
  Saturation5/1 -> Gain/1, Product5/2
  Divide3/1 -> Sum1/2
  Product6/1 -> Sum/1  "Current Request (0-75amps)"
  Constant28/1 -> Switch3/3
  Square/1 -> Product3/1
  Saturation2/1 -> Subtract2/1  "Exponential Throttle Map"
  Sum3/1 -> Out1/1, Scope11/1
  Constant16/1 -> Less Than/2  "Max Battery temp"
  GreaterThan3/1 -> Switch3/2
  Constant6/1 -> Subtract1/1  "Minimum Throttle Percentage"
  Constant9/1 -> Product3/2
  Add2/1 -> Saturation1/1
  Wheel Speed (m/s)/1 -> Product1/1  "Speed (m/s)"
  AND3/1 -> Scope3/1, AND/2  "Battery Logic"
  Divide/1 -> Divide4/1
  Compare To Constant/1 -> AND/1, Scope1/1
  Sum/1 -> Saturation5/1
  Constant18/1 -> Less Than1/2  "Max Battery SOC"
  Constant7/1 -> Subtract1/2  "Intial distance"
  AND2/1 -> AND3/2
  Memory1/1 -> Sum/2
  AND1/1 -> AND3/1
  Constant2/1 -> Product1/2
  Data Store Read1/1 -> Minus/2, Product7/1, Relay/1
  Constant4/1 -> Subtract/1  "Min Regen Percentage"
  Less Than1/1 -> AND2/2
  Minus/1 -> Divide/1  "Voltage Threshold to overcharge"
  GreaterThan/1 -> AND1/1
  Scale/1 -> Product4/2
  Sum1/1 -> Saturation3/1
  Divide1/1 -> Product2/2  "Slope"
  Constant15/1 -> Divide/2  "Battery Internal Resistance"
  Switch2/1 -> Data Store Write/1, Product7/2  "Charge Current"
  Product4/1 -> Scope/1, Switch1/3, GreaterThan2/1  "Requested Charge Current"
  Product2/1 -> Add3/2
  Relay/1 -> Switch2/2, Scope7/1
  Battery Temp/1 -> GreaterThan/1, Less Than/1  "Battery Temp"
  Switch1/1 -> Switch2/1, Scope8/1
  Less Than/1 -> AND1/2
  Gain/1 -> Data Store Write1/1
  Divide4/1 -> GreaterThan2/2, Switch1/1, Scope9/1  "Maximum Permissable Charge Current"
  Gain3/1 -> Product6/1
  IC1/1 -> Divide2/2
  Data Store Read2/1 -> Divide3/1
  Constant/1 -> Divide3/2
  Discrete PID Controller1/1 -> Memory1/1
  Divide2/1 -> Discrete PID Controller1/1  "Current Error"
  Data Store Read3/1 -> Divide5/1
  Divide5/1 -> Gain3/1
  Data Store Read/1 -> Divide5/2, Moving Average/1
  Gain2/1 -> Product6/2

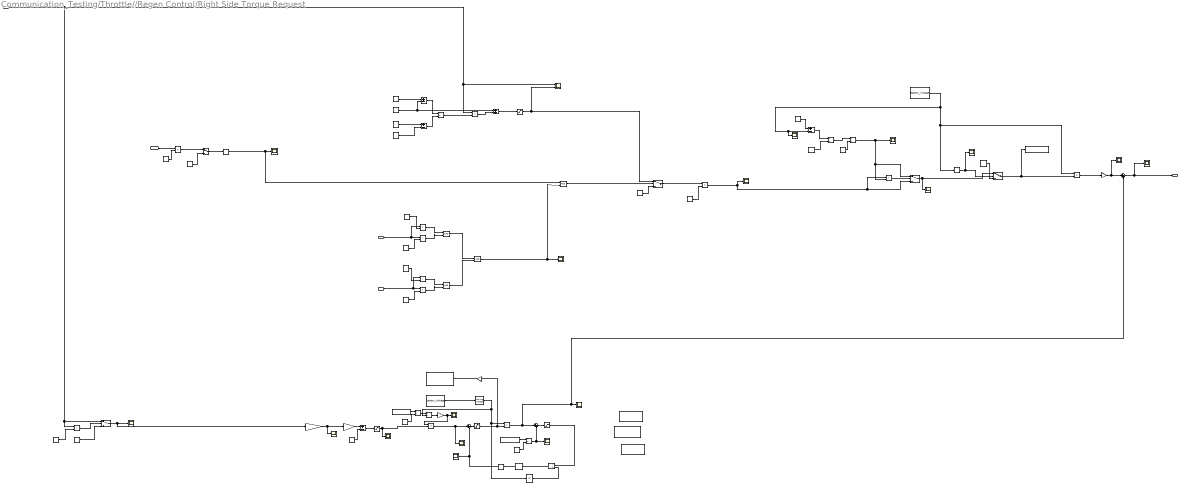
== system Communication_Testing/Throttle//Regen Control/Right Side Torque Request ==
  note: Maps 0.1 rather then percentage
  note: Halveing as this is the permissable for left/right side inverter
  note: If Conditions are not fulfilled charge current is set to zero
  note: Throttle pedal to regen percentage request
  note: Power Limiting to maintatin Power Limit of Less then 80 Kw
  note: throttle output enabled when less then 20% actuation, this will be used for regen
  note: If Battery Voltage greater then 590 Charge Current is set to zero
  note: Speed Threshold, Regen enabled above 5km/h
  note: Max Charge Current, Regen is scalled 0-100%. Current wants to be 0 -130 amps, therfore scale by 1.3. 600V*130amps = 70kw, Then divide by two for left and right motor Control
  note: Hysterisies Control
  note: Inverting as this is a discharge current
  note: Battery Checks
  note: This is the threshold for when drive torque is requested, Regen is requested for less then 20%, and throttle is applied for greater then 22%, This gives a 2% deadband
  note: If Requested Charge current is greater then permissable charge current then switch to permisable
  In1 : Inport
  Wheel Speed (m/s) : Inport  Port=2
  Battery Temp : Inport  Port=3
  Battery SOC : Inport  Port=4
  AND{,1..3} (4 alike) : Logic  IconShape=distinctive  AllPortsSameDT=off  OutDataTypeStr=boolean
  Add3 : Sum
  Compare To Constant : simulink/Logic and Bit Operations/Compare To Constant  relop=>  const=5  OutDataTypeStr=boolean
  Constant : Constant  Value=2
  Constant1 : Constant  Value=2
  Constant{7,11,21,28} (4 alike) : Constant  Value=0
  Constant12 : Constant  Value=6
  Constant15 : Constant  Value=0.01
  Constant16 : Constant  Value=50
  Constant17 : Constant  Value=10
  Constant18 : Constant  Value=90
  Constant19 : Constant  Value=5
  Constant2 : Constant  Value=3.6
  Constant20 : Constant  Value=580
  Constant26 : Constant  Value=2
  Constant27 : Constant  Value=22
  Constant3 : Constant  Value=0.22
  Constant4 : Constant  Value=10
  Constant5 : Constant  Value=100
  Constant6 : Constant  Value=20
  Data Store Memory2 : DataStoreMemory  DataStoreName=Right_Sim_Regen_Current  WriteAfterWriteMsg=warning  ShowAdditionalParam=off
  Data Store Memory3 : DataStoreMemory  DataStoreName=Left_Sim_Discharge_Current  WriteAfterWriteMsg=warning  ShowAdditionalParam=off
  Data Store Memory4 : DataStoreMemory  DataStoreName=Left_Sim_Regen_Current  WriteAfterWriteMsg=warning  ShowAdditionalParam=off
  Data Store Read : DataStoreRead  DataStoreName=Battery_Voltage  IndexOptions=Index vector (dialog)  Indices=1  OutputSizes=1
  Data Store Read1 : DataStoreRead  DataStoreName=Battery_Voltage  IndexOptions=Index vector (dialog)  Indices=1  OutputSizes=1
  Data Store Read2 : DataStoreRead  DataStoreName=Global_Power_Limit  IndexOptions=Index vector (dialog)  Indices=1  OutputSizes=1
  Data Store Read3 : DataStoreRead  DataStoreName=Global_Power_Limit  IndexOptions=Index vector (dialog)  Indices=1  OutputSizes=1
  Data Store Write : DataStoreWrite  DataStoreName=Right_Sim_Discharge_Current  IndexOptions=Index vector (dialog)  Indices=1  OutputSizes=1
  Data Store Write1 : DataStoreWrite  DataStoreName=Right_Sim_Regen_Current  IndexOptions=Index vector (dialog)  Indices=1  OutputSizes=1
  Discrete PID Controller1 : slpidlib/PID Controller  Controller=PID  Form=Parallel  TimeDomain=Discrete-time  UseExternalTs=off  SampleTime=-1  IntegratorMethod=Forward Euler  FilterMethod=Forward Euler  ControllerParametersSource=internal  P=0.000544217300579932  I=0.544217300579932  UseKiTs=on  D=0  UseExternalDerivativeSource=off  N=100  UseFilter=on  TunerSelectOption=Transfer Function Based (PID Tuner App)  InitialConditionSource=internal  InitialConditionForIntegrator=0  InitialConditionForFilter=0  DifferentiatorICPrevScaledInput=0  ExternalReset=none  TrackingMode=off  Kt=1  LimitOutput=off  SatLimitsSource=internal  UpperSaturationLimit=inf  LowerSaturationLimit=-inf  LinearizeAsGain=off  AntiWindupMode=none  Kb=1  LimitIntegrator=off  UpperIntegratorSaturationLimit=inf  LowerIntegratorSaturationLimit=-inf  POutMin=[]  POutMax=[]  IOutMin=[]  IOutMax=[]  DOutMin=[]  DOutMax=[]  NOutMin=[]  NOutMax=[]  SumOutMin=[]  SumOutMax=[]  SaturationOutMin=[]  SaturationOutMax=[]  PParamMin=[]  PParamMax=[]  IParamMin=[]  IParamMax=[]  DParamMin=[]  DParamMax=[]  NParamMin=[]  NParamMax=[]  KbParamMin=[]  KbParamMax=[]  KtParamMin=[]  KtParamMax=[]  KbOutMin=[]  KbOutMax=[]  KtOutMin=[]  KtOutMax=[]  IntegratorOutMin=[]  IntegratorOutMax=[]  FilterOutMin=[]  FilterOutMax=[]  SumI1OutMin=[]  SumI1OutMax=[]  SumI2OutMin=[]  SumI2OutMax=[]  SumI3OutMin=[]  SumI3OutMax=[]  SumI4OutMin=[]  SumI4OutMax=[]  SumDOutMin=[]  SumDOutMax=[]  DifferentiatorOutMin=[]  DifferentiatorOutMax=[]  FilterDiffOutCoefMin=[]  FilterDiffOutCoefMax=[]  ReciprocalOutMin=[]  ReciprocalOutMax=[]  SumDenOutMin=[]  SumDenOutMax=[]  SumNumOutMin=[]  SumNumOutMax=[]  DivideOutMin=[]  DivideOutMax=[]  UdiffTsProdOutMin=[]  UdiffTsProdOutMax=[]  NTsProdOutMin=[]  NTsProdOutMax=[]  UintegralTsProdOutMin=[]  UintegralTsProdOutMax=[]  UngainTsProdOutMin=[]  UngainTsProdOutMax=[]  ClampingZeroOutDataTypeStr=Inherit: Inherit via back propagation  ClampingZeroOutMin=[]  ClampingZeroOutMax=[]  FilterDenConstantOutDataTypeStr=Inherit: Inherit via back propagation  FilterDenConstantOutMin=[]  FilterDenConstantOutMax=[]  PCopyOutDataTypeStr=Inherit: Inherit via back propagation  PCopyOutMin=[]  PCopyOutMax=[]  NCopyOutDataTypeStr=Inherit: Inherit via back propagation  NCopyOutMin=[]  NCopyOutMax=[]  IntegratorContinuousStateAttributes=''  IntegratorStateMustResolveToSignalObject=off  IntegratorRTWStateStorageClass=Auto  FilterContinuousStateAttributes=''  FilterStateMustResolveToSignalObject=off  FilterRTWStateStorageClass=Auto  ParallelPVariant=InternalParameters  IdealPVariant=Disabled  IVariant=InternalParameters  DVariant=InternalParameters  IntegratorVariant=Discrete  SatVariant=Disabled  AWVariant=Passthrough  PCopyVariant=Disabled  TRVariant=Disabled  FdbkBlocksVariant=Forward  IdealPFdbkVariant=Disabled  SatFdbkVariant=Disabled  DerivativeFilterVariant=ForwardEulerFilter  NVariant=InternalParameters  NCopyVariant=Disabled  FilterICVariant=InternalICsFilter  IntegratorICVariant=InternalICs  ExternalResetVariant=Disabled  TRSumVariant=Passthrough  SumFdbkVariant=Disabled  SumVariant=Sum_PID  TsampFilterVariant=InternalTs  TsampNgainVariant=Passthrough  TsampIntegralVariant=Disabled_SignalSpec  ExternalSaturationOutDataTypeStr=Inherit: Same as second input  DerivativeSourceVariant=ErrorSignal
      settings: LibrarySourceBlock=simulink/Discrete/Discrete PID Controller
  Divide{,1..6} (7 alike) : Product  Inputs=*/
  Gain : Gain  Gain=-1
  Gain1 : Gain  Gain=-1
  Gain2 : Gain  Gain=1/100
  Gain3 : Gain  Gain=1.1
  Gain4 : Gain  Gain=1.22
  GreaterThan{,1..3} (4 alike) : RelationalOperator  Operator=>  OutDataTypeStr=boolean  RndMeth=Simplest  InputSameDT=off
  IC2 : InitialCondition  Value=600
  Less Than : RelationalOperator  Operator=<  OutDataTypeStr=boolean  RndMeth=Simplest  InputSameDT=off
  Less Than1 : RelationalOperator  Operator=<  OutDataTypeStr=boolean  RndMeth=Simplest  InputSameDT=off
  Manual Switch1 : ManualSwitch
  Memory1 : Memory  InitialCondition=14  InheritSampleTime=on
  Minus : Sum  Inputs=+-
  Moving Average : dspstat3/Moving Average  Method=Sliding window  ForgettingFactorPort=off  SpecifyWindowLength=on  WindowLength=10  OverlapLength=9  AllowArbitraryInputLength=off  ForgettingFactor=0.9  SimulateUsing=Interpreted execution
  Product{1..2,4..7} (6 alike) : Product
  Relay : Relay  OnSwitchValue=590  OffSwitchValue=585  OnOutputValue=0  OffOutputValue=1
  Saturation : Saturate  UpperLimit=100  LowerLimit=0
  Saturation1 : Saturate  UpperLimit=1  LowerLimit=0
  Saturation3 : Saturate  UpperLimit=inf  LowerLimit=0
  Saturation5 : Saturate  UpperLimit=inf  LowerLimit=0
  Scale : Constant  Value=0.65
  Scope{,1,3..17} (17 alike) : Scope
  Scope2 : Scope  NumInputPorts=2
  Subtract : Sum  Inputs=+-
  Subtract1 : Sum  Inputs=+-
  Subtract2 : Sum  Inputs=+-
  Sum : Sum  Inputs=|+-
  Sum1 : Sum  Inputs=|+-
  Sum3 : Sum  Inputs=|++
  Switch : Switch  Criteria=u2 > Threshold  SaturateOnIntegerOverflow=off  InputSameDT=off
  Switch1 : Switch  Criteria=u2 > Threshold  SaturateOnIntegerOverflow=off  InputSameDT=off
  Switch2 : Switch  Criteria=u2 > Threshold  Threshold=0.5  SaturateOnIntegerOverflow=off  InputSameDT=off
  Switch3 : Switch  Criteria=u2 > Threshold  SaturateOnIntegerOverflow=off  InputSameDT=off
  Out1 : Outport
  wires:
  Constant26/1 -> Divide4/2
  AND/1 -> Switch/2
  Add3/1 -> Saturation/1  "Regen Request"
  GreaterThan2/1 -> Switch1/2
  Constant12/1 -> Manual Switch1/2
  GreaterThan1/1 -> AND2/1
  Constant21/1 -> Switch2/3
  In1/1 -> Switch3/1, GreaterThan3/1, Product2/1, Scope2/1  "Throttle Pedal"
  Constant11/1 -> Switch/3
  Switch3/1 -> Gain2/1, Scope14/1  "Throttle Percentage > 20"
  Product5/1 -> Sum3/2, Scope5/1, Sum1/1  "Requested Discharge Power"
  Saturation/1 -> Switch/1, Scope2/2  "Linear Regen Map"
  Switch/1 -> Product4/1  "Requested Charge Current"
  Constant27/1 -> GreaterThan3/2
  Constant20/1 -> Minus/1  "Max Battery Voltage using Regen"
  Constant5/1 -> Subtract/2, Add3/1  "Max Regen Percentage"
  Constant19/1 -> GreaterThan1/2  "Min Battery SOC"
  Product7/1 -> Gain1/1  "Requested Charge Power"
  Subtract/1 -> Divide1/1
  Battery SOC/1 -> GreaterThan1/1, Less Than1/1  "Battery State of Charge"
  Moving Average/1 -> IC2/1, Product5/1, Divide5/2
  Divide2/1 -> Discrete PID Controller1/1  "Current Error"
  Saturation3/1 -> Divide2/1  "Power Error"
  Manual Switch1/1 -> Compare To Constant/1
  Product1/1 -> Manual Switch1/1  "Speed (km/h)"
  Subtract1/1 -> Divide1/2
  Constant17/1 -> GreaterThan/2  "Min Battery Temp"
  Saturation5/1 -> Gain/1, Product5/2
  Divide3/1 -> Scope6/1, Sum1/2
  Product6/1 -> Sum/1, Scope10/1  "Current Request (0-75amps)"
  Constant28/1 -> Switch3/3
  Sum3/1 -> Out1/1, Scope11/1
  Constant16/1 -> Less Than/2  "Max Battery temp"
  GreaterThan3/1 -> Switch3/2
  Constant6/1 -> Subtract1/1  "Minimum Throttle Percentage"
  Wheel Speed (m/s)/1 -> Product1/1  "Speed (m/s)"
  AND3/1 -> Scope3/1, AND/2  "Battery Logic"
  Divide/1 -> Divide4/1
  Compare To Constant/1 -> AND/1, Scope1/1
  Sum/1 -> Saturation5/1
  Constant18/1 -> Less Than1/2  "Max Battery SOC"
  Constant7/1 -> Subtract1/2  "Intial distance"
  AND2/1 -> AND3/2
  Memory1/1 -> Sum/2, Scope12/1
  AND1/1 -> AND3/1
  Constant2/1 -> Product1/2
  Data Store Read1/1 -> Scope15/1, Minus/2, Product7/1, Relay/1
  Constant4/1 -> Subtract/1  "Min Regen Percentage"
  Less Than1/1 -> AND2/2
  Minus/1 -> Divide/1  "Voltage Threshold to overcharge"
  GreaterThan/1 -> AND1/1
  Scale/1 -> Product4/2
  Sum1/1 -> Saturation3/1
  Divide1/1 -> Product2/2  "Slope"
  Constant15/1 -> Divide/2  "Battery Internal Resistance"
  Switch2/1 -> Data Store Write1/1, Product7/2  "Charge Current"
  Product4/1 -> Scope/1, Switch1/3, GreaterThan2/1  "Requested Charge Current"
  Product2/1 -> Add3/2
  Relay/1 -> Switch2/2, Scope7/1
  Battery Temp/1 -> GreaterThan/1, Less Than/1  "Battery Temp"
  Switch1/1 -> Switch2/1, Scope8/1
  Less Than/1 -> AND1/2
  Gain/1 -> Data Store Write/1
  Divide4/1 -> GreaterThan2/2, Switch1/1, Scope9/1  "Maximum Permissable Charge Current"
  Gain3/1 -> Scope16/1, Product6/1
  IC2/1 -> Divide2/2
  Data Store Read2/1 -> Divide3/1
  Constant/1 -> Divide3/2
  Discrete PID Controller1/1 -> Memory1/1
  Gain1/1 -> Scope13/1, Sum3/1
  Data Store Read/1 -> Moving Average/1
  Data Store Read3/1 -> Divide6/1
  Divide5/1 -> Gain3/1
  Constant1/1 -> Divide6/2
  Divide6/1 -> Divide5/1
  Subtract2/1 -> Saturation1/1
  Gain2/1 -> Gain4/1, Scope4/1
  Constant3/1 -> Subtract2/2
  Saturation1/1 -> Scope17/1, Product6/2
  Gain4/1 -> Subtract2/1
